simulink subsystem "GCAS"  (R2023b)
settings: Solver=VariableStepAuto  StartTime=0.0  StopTime=10.0  RelTol=1e-3
undefined symbols (not defined in the file): Altitudes, faces, Latitudes, Longitudes, spacing_in_latitude, spacing_in_longitude, vertices
libraries: simulink x3, simulink_extras x1
settings Model: Creator=cyber  LastModifiedBy=cyber

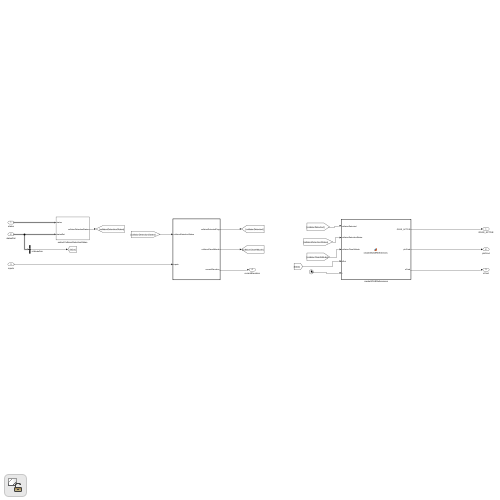
[thumbnail: Simulink's stored preview of the top-level diagram]
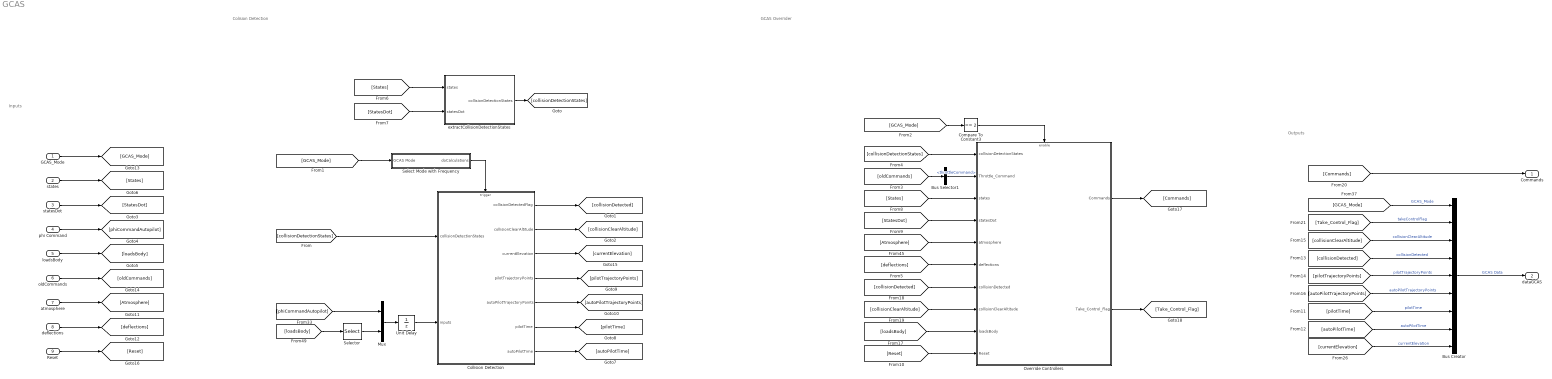
== system GCAS ==
  note: Inputs
  note: Outputs
  note: Colision Detection
  note: GCAS Overrider
  GCAS_Mode : Inport
  states : Inport  Port=2
  statesDot : Inport  Port=3
  phi Command : Inport  Port=4
  loadsBody : Inport  Port=5
  oldCommands : Inport  Port=6
  atmosphere : Inport  Port=7
  deflections : Inport  Port=8
  Reset : Inport  Port=9
  Bus Creator : BusCreator  Inputs=9
  Bus Selector1 : BusSelector  OutputSignals=throttleCommand
  Collision Detection : Subsystem  TreatAsAtomicUnit=on  SystemSampleTime=0.5
  Compare To Constant3 : simulink/Logic and Bit Operations/Compare To Constant  relop===  const=2  OutDataTypeStr=boolean
  Mux : Mux  Inputs=2
  Override Controllers : Subsystem
  Select Mode with Frequency : Subsystem
  Selector : Selector  InputPortWidth=3  IndexOptions=Index vector (dialog)  Indices=[3]  OutputSizes=1
  Unit Delay : UnitDelay  InitialCondition=[0,1]  SampleTime=-1  HasFrameUpgradeWarning=on
  extractCollisionDetectionStates : Subsystem
  Commands : Outport
  dataGCAS : Outport  Port=2
  wires:
  extractCollisionDetectionStates/1(collisionDetectionStates) -> [collisionDetectionStates]
  [collisionDetectionStates] -> Collision Detection/1(collisionDetectionStates)
  Collision Detection/1(collisionDetectedFlag) -> [collisionDetected]
  Collision Detection/2(collisionClearAltitude) -> [collisionClearAltitude]
  Collision Detection/3(currentElevation) -> [currentElevation]
  Collision Detection/4(pilotTrajectoryPoints) -> [pilotTrajectoryPoints]
  Collision Detection/5(autoPilotTrajectoryPoints) -> [autoPilotTrajectoryPoints]
  Collision Detection/7(autoPilotTime) -> [autoPilotTime]
  Collision Detection/6(pilotTime) -> [pilotTime]
  Unit Delay/1 -> Collision Detection/2(inputs)
  Mux/1 -> Unit Delay/1
  [phiCommandAutopilot] -> Mux/1
  [loadsBody] -> Selector/1
  Selector/1 -> Mux/2
  phi Command/1 -> [phiCommandAutopilot]
  loadsBody/1 -> [loadsBody]
  GCAS_Mode/1 -> [GCAS_Mode]
  oldCommands/1 -> [oldCommands]
  Override Controllers/1(Commands) -> [Commands]
  [GCAS_Mode] -> Compare To Constant3/1
  Compare To Constant3/1 -> Override Controllers/Enable
  [oldCommands] -> Bus Selector1/1
  Bus Selector1/1 -> Override Controllers/2(Throttle_Command)  "<throttleCommand>"
  [collisionDetectionStates] -> Override Controllers/1(collisionDetectionStates)
  states/1 -> [States]
  statesDot/1 -> [StatesDot]
  [States] -> extractCollisionDetectionStates/1(states)
  [StatesDot] -> extractCollisionDetectionStates/2(statesDot)
  [States] -> Override Controllers/3(states)
  [StatesDot] -> Override Controllers/4(statesDot)
  atmosphere/1 -> [Atmosphere]
  [Atmosphere] -> Override Controllers/5(atmosphere)
  Reset/1 -> [Reset]
  deflections/1 -> [deflections]
  [Reset] -> Override Controllers/10(Reset)
  [deflections] -> Override Controllers/6(deflections)
  [pilotTrajectoryPoints] -> Bus Creator/5  "pilotTrajectoryPoints"
  [Take_Control_Flag] -> Bus Creator/2  "takeControlFlag"
  [autoPilotTrajectoryPoints] -> Bus Creator/6  "autoPilotTrajectoryPoints"
  [collisionClearAltitude] -> Bus Creator/3  "collisionClearAltitude"
  [pilotTime] -> Bus Creator/7  "pilotTime"
  [currentElevation] -> Bus Creator/9  "currentElevation"
  [autoPilotTime] -> Bus Creator/8  "autoPilotTime"
  [collisionDetected] -> Bus Creator/4  "collisionDetected"
  Bus Creator/1 -> dataGCAS/1  "GCAS Data"
  [GCAS_Mode] -> Bus Creator/1  "GCAS_Mode"
  [collisionDetected] -> Override Controllers/7(collisionDetected)
  [collisionClearAltitude] -> Override Controllers/8(collisionClearAltitude)
  [Commands] -> Commands/1
  Override Controllers/2(Take_Control_Flag) -> [Take_Control_Flag]
  [loadsBody] -> Override Controllers/9(loadsBody)
  [GCAS_Mode] -> Select Mode with Frequency/1(GCAS Mode)
  Select Mode with Frequency/1(doCalculations) -> Collision Detection/Trigger

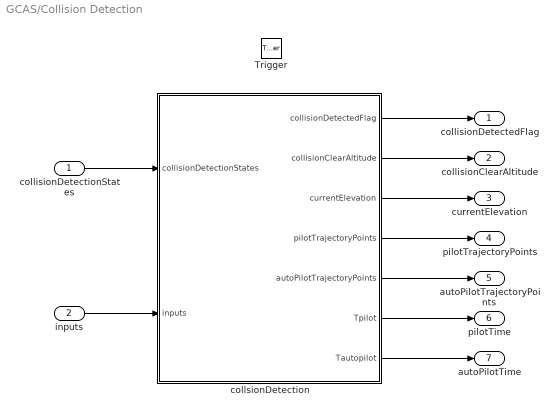
== system GCAS/Collision Detection ==
  collisionDetectionStates : Inport
  inputs : Inport  Port=2
  Trigger : TriggerPort  VariantControl=(inherit)  InitialTriggerSignalState=zero  PortDimensions=1
  collsionDetection : MATLAB Function  TreatAsAtomicUnit=on
  collisionDetectedFlag : Outport
  collisionClearAltitude : Outport  Port=2
  currentElevation : Outport  Port=3
  pilotTrajectoryPoints : Outport  Port=4
  autoPilotTrajectoryPoints : Outport  Port=5
  pilotTime : Outport  Port=6
  autoPilotTime : Outport  Port=7
  wires:
  collsionDetection/6(Tpilot) -> pilotTime/1
  collsionDetection/7(Tautopilot) -> autoPilotTime/1
  collsionDetection/5(autoPilotTrajectoryPoints) -> autoPilotTrajectoryPoints/1
  collsionDetection/4(pilotTrajectoryPoints) -> pilotTrajectoryPoints/1
  collsionDetection/3(currentElevation) -> currentElevation/1
  inputs/1 -> collsionDetection/2(inputs)
  collsionDetection/2(collisionClearAltitude) -> collisionClearAltitude/1
  collisionDetectionStates/1 -> collsionDetection/1(collisionDetectionStates)
  collsionDetection/1(collisionDetectedFlag) -> collisionDetectedFlag/1

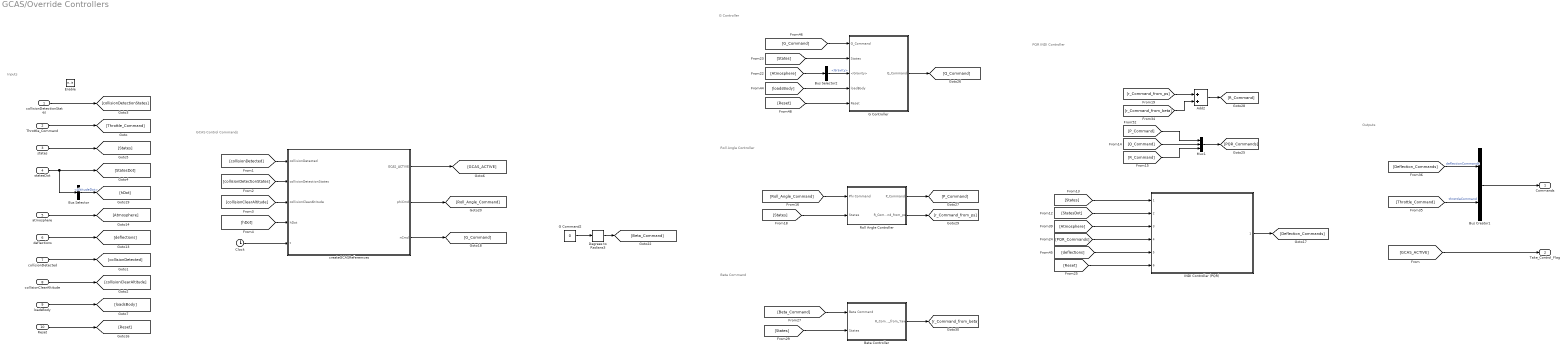
== system GCAS/Override Controllers ==
  note: Inputs
  note: Beta Command
  note: PQR INDI Controller
  note: Roll Angle Controller
  note: G Controller
  note: GCAS Control Commands
  note: Outputs
  collisionDetectionStates : Inport
  Throttle_Command : Inport  Port=2
  states : Inport  Port=3
  statesDot : Inport  Port=4
  atmosphere : Inport  Port=5
  deflections : Inport  Port=6
  collisionDetected : Inport  Port=7
  collisionClearAltitude : Inport  Port=8
  loadsBody : Inport  Port=9
  Reset : Inport  Port=10
  Enable : EnablePort
  Add2 : Sum
  Beta Controller : Subsystem  TreatAsAtomicUnit=on
  Bus Creator1 : BusCreator  Inputs=2
  Bus Selector : BusSelector  OutputSignals=AltitudeDot
  Bus Selector2 : BusSelector  OutputSignals=Gravity
  Clock : Clock
  Degrees to Radians3 : simulink_extras/Transformations/Degrees to Radians
  G Command2 : Constant  Value=0
  G Controller : Subsystem  TreatAsAtomicUnit=on
  INDI Controller (PQR) : Subsystem  ReferencedSubsystem=INDI_Controller_PQR
  Mux1 : Mux  Inputs=3
  Roll Angle Controller : Subsystem  TreatAsAtomicUnit=on
  createGCASReferemces : MATLAB Function  TreatAsAtomicUnit=on
  Commands : Outport
  Take_Control_Flag : Outport  Port=2
  wires:
  loadsBody/1 -> [loadsBody]
  [GCAS_ACTIVE] -> Take_Control_Flag/1
  collisionClearAltitude/1 -> [collisionClearAltitude]
  collisionDetected/1 -> [collisionDetected]
  Bus Selector/1 -> [hDot]  "<AltitudeDot>"
  deflections/1 -> [deflections]
  Reset/1 -> [Reset]
  atmosphere/1 -> [Atmosphere]
  states/1 -> [States]
  statesDot/1 -> Bus Selector/1, [StatesDot]
  collisionDetectionStates/1 -> [collisionDetectionStates]
  Throttle_Command/1 -> [Throttle_Command]
  createGCASReferemces/2(phiCmd) -> [Roll_Angle_Command]
  [r_Command_from_ps] -> Add2/1
  [States] -> Beta Controller/2(States)
  [Atmosphere] -> INDI Controller (PQR)/3
  Degrees to Radians3/1 -> [Beta_Command]
  G Command2/1 -> Degrees to Radians3/1
  [PQR_Commands] -> INDI Controller (PQR)/4
  [G_Command] -> G Controller/1(G_Command)
  [r_Command_from_beta] -> Add2/2
  [R_Command] -> Mux1/3
  [States] -> INDI Controller (PQR)/1
  [States] -> G Controller/2(States)
  [P_Command] -> Mux1/1
  [Beta_Command] -> Beta Controller/1(Beta Command)
  [collisionDetectionStates] -> createGCASReferemces/2(collisionDetectionStates)
  G Controller/1(Q_Command) -> [Q_Command]
  Beta Controller/1(R_Command_from_Yaw) -> [r_Command_from_beta]
  Add2/1 -> [R_Command]
  INDI Controller (PQR)/1 -> [Deflection_Commands]
  [Q_Command] -> Mux1/2
  [Atmosphere] -> Bus Selector2/1
  Roll Angle Controller/2(R_Command_from_ps) -> [r_Command_from_ps]
  Bus Selector2/1 -> G Controller/3(<Gravity>)  "<Gravity>"
  [hDot] -> createGCASReferemces/4(hDot)
  Mux1/1 -> [PQR_Commands]
  [collisionDetected] -> createGCASReferemces/1(collisionDetected)
  createGCASReferemces/1(GCAS_ACTIVE) -> [GCAS_ACTIVE]
  createGCASReferemces/3(nCmd) -> [G_Command]
  [loadsBody] -> G Controller/4(loadBody)
  [deflections] -> INDI Controller (PQR)/5
  [Deflection_Commands] -> Bus Creator1/1  "deflectionCommands"
  [Reset] -> INDI Controller (PQR)/6
  Roll Angle Controller/1(P_Command) -> [P_Command]
  [Reset] -> G Controller/5(Reset)
  [States] -> Roll Angle Controller/2(States)
  [collisionClearAltitude] -> createGCASReferemces/3(collisionClearAltitude)
  [StatesDot] -> INDI Controller (PQR)/2
  [Throttle_Command] -> Bus Creator1/2  "throttleCommand"
  Clock/1 -> createGCASReferemces/5(t)
  [Roll_Angle_Command] -> Roll Angle Controller/1(Phi Command)
  Bus Creator1/1 -> Commands/1

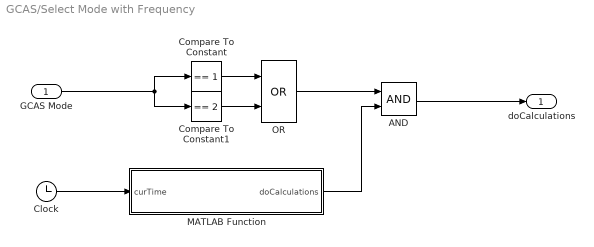
== system GCAS/Select Mode with Frequency ==
  GCAS Mode : Inport
  AND : Logic  AllPortsSameDT=off  OutDataTypeStr=boolean
  Clock : Clock
  Compare To Constant : simulink/Logic and Bit Operations/Compare To Constant  relop===  const=1  OutDataTypeStr=boolean
  Compare To Constant1 : simulink/Logic and Bit Operations/Compare To Constant  relop===  const=2  OutDataTypeStr=boolean
  MATLAB Function : MATLAB Function  TreatAsAtomicUnit=on
  OR : Logic  Operator=OR  AllPortsSameDT=off  OutDataTypeStr=boolean
  doCalculations : Outport
  wires:
  MATLAB Function/1(doCalculations) -> AND/2
  Clock/1 -> MATLAB Function/1(curTime)
  AND/1 -> doCalculations/1
  OR/1 -> AND/1
  GCAS Mode/1 -> Compare To Constant1/1, Compare To Constant/1
  Compare To Constant/1 -> OR/1
  Compare To Constant1/1 -> OR/2

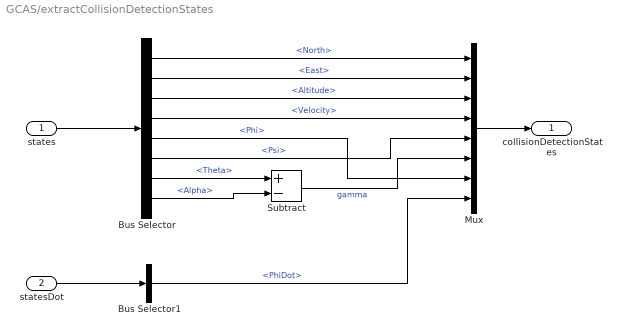
== system GCAS/extractCollisionDetectionStates ==
  states : Inport
  statesDot : Inport  Port=2
  Bus Selector : BusSelector  OutputSignals=North,East,Altitude,Velocity,Phi,Psi,Theta,Alpha
  Bus Selector1 : BusSelector  OutputSignals=PhiDot
  Mux : Mux  Inputs=8
  Subtract : Sum  Inputs=+-
  collisionDetectionStates : Outport
  wires:
  Mux/1 -> collisionDetectionStates/1
  Subtract/1 -> Mux/6  "gamma"
  Bus Selector/4 -> Mux/4  "<Velocity>"
  Bus Selector/2 -> Mux/2  "<East>"
  states/1 -> Bus Selector/1
  Bus Selector1/1 -> Mux/8  "<PhiDot>"
  Bus Selector/6 -> Mux/5  "<Psi>"
  Bus Selector/8 -> Subtract/2  "<Alpha>"
  statesDot/1 -> Bus Selector1/1
  Bus Selector/5 -> Mux/7  "<Phi>"
  Bus Selector/3 -> Mux/3  "<Altitude>"
  Bus Selector/1 -> Mux/1  "<North>"
  Bus Selector/7 -> Subtract/1  "<Theta>"

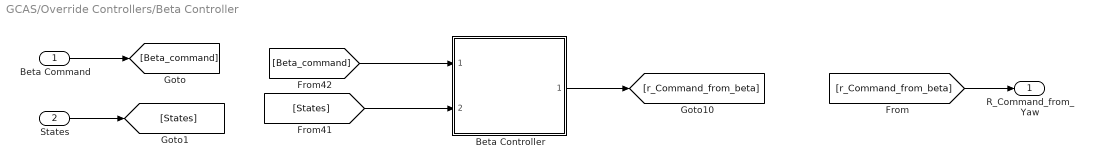
== system GCAS/Override Controllers/Beta Controller ==
  Beta Command : Inport
  States : Inport  Port=2
  Beta Controller : Subsystem  ReferencedSubsystem=Beta_Controller
  R_Command_from_Yaw : Outport
  wires:
  Beta Controller/1 -> [r_Command_from_beta]
  [States] -> Beta Controller/2
  [Beta_command] -> Beta Controller/1
  Beta Command/1 -> [Beta_command]
  [r_Command_from_beta] -> R_Command_from_Yaw/1
  States/1 -> [States]

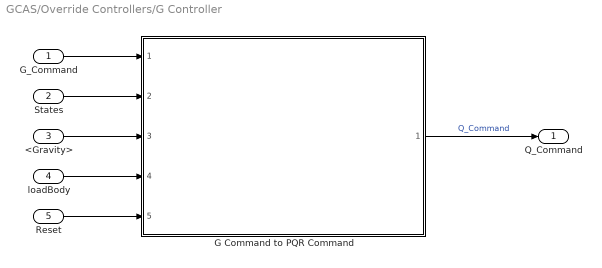
== system GCAS/Override Controllers/G Controller ==
  G_Command : Inport
  States : Inport  Port=2
  <Gravity> : Inport  Port=3
  loadBody : Inport  Port=4
  Reset : Inport  Port=5
  G Command to PQR Command : Subsystem  ReferencedSubsystem=G_Command_to_PQR_Command
  Q_Command : Outport
  wires:
  Reset/1 -> G Command to PQR Command/5
  States/1 -> G Command to PQR Command/2
  G_Command/1 -> G Command to PQR Command/1
  <Gravity>/1 -> G Command to PQR Command/3
  loadBody/1 -> G Command to PQR Command/4
  G Command to PQR Command/1 -> Q_Command/1  "Q_Command"

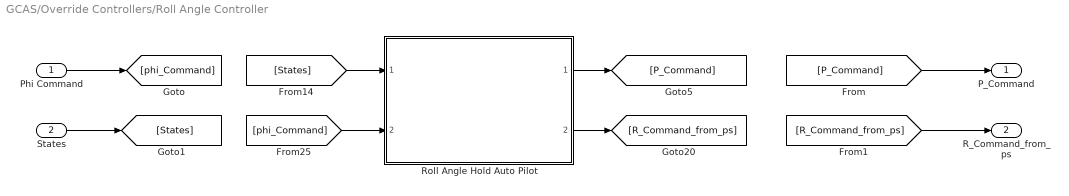
== system GCAS/Override Controllers/Roll Angle Controller ==
  Phi Command : Inport
  States : Inport  Port=2
  "Roll Angle Hold Auto Pilot " : Subsystem  ReferencedSubsystem=Roll_Angle_Hold_Auto_Pilot
  P_Command : Outport
  R_Command_from_ps : Outport  Port=2
  wires:
  States/1 -> [States]
  [R_Command_from_ps] -> R_Command_from_ps/1
  [P_Command] -> P_Command/1
  Phi Command/1 -> [phi_Command]
  [States] -> "Roll Angle Hold Auto Pilot "/1
  [phi_Command] -> "Roll Angle Hold Auto Pilot "/2
  "Roll Angle Hold Auto Pilot "/1 -> [P_Command]
  "Roll Angle Hold Auto Pilot "/2 -> [R_Command_from_ps]

== matlab function GCAS/Collision Detection/collsionDetection ==
  data: collisionDetectionStates input; collisionDetectedFlag output size=1; inputs input; Latitudes parameter; Longitudes parameter; Altitudes parameter; spacing_in_latitude parameter; spacing_in_longitude parameter; vertices parameter; faces parameter; collisionClearAltitude output; currentElevation output; pilotTrajectoryPoints output; autoPilotTrajectoryPoints output; Tpilot output; Tautopilot output
function [collisionDetectedFlag,collisionClearAltitude, currentElevation, pilotTrajectoryPoints, autoPilotTrajectoryPoints, Tpilot,Tautopilot]  = collisionDetection(collisionDetectionStates, inputs, Latitudes, Longitudes, Altitudes, spacing_in_latitude, spacing_in_longitude, vertices, faces)
    
    coder.extrinsic("visualizeTraj")
    visualize_traj = false;
    x = collisionDetectionStates(1); 
    y = collisionDetectionStates(2); 
    h = collisionDetectionStates(3);
    V = collisionDetectionStates(4);
    psi = collisionDetectionStates(5); 
    gamma = collisionDetectionStates(6); 
    phi = collisionDetectionStates(7);
    phiDot = collisionDetectionStates(8); 
    
    phiPilot = inputs(1); 
    nGPilot = inputs(2);
    Tpilot = 1;
    
    % define reference latitude longitude altitude
    lat0 = 41.10068727249253;
    lon0 = 29.024573561608477;
    h0 = 0;

    g = 9.81; % gravitational constant
    dt = 0.1; 
    T = 20;
    ts = 2.25; % Roll dynamics settling time
    OS = 1.4030 / 100; % Roll dynamics overshoot value
    zeta = - log(OS) / sqrt(pi^2+ log(OS)^2); % roll dynamics damping ratio
    wn = 4/(zeta*ts); % roll dynamics natural freq
    tsG = 2.0; % G controller settling time
    zetaG = 1; % G controller dampling ratio
    wnG = 4 / (zetaG*tsG); % G controller natural frequency

    N = floor(T/dt);
    t_array = 0:dt:T;
    states_list = zeros(N+1, 6);
    inputs_list = zeros(N+1,2);
    states_list(1,:) = [x,y,h,psi, gamma, phi];
    inputs_list(1,:) = [phiPilot, nGPilot];
    phiCmd = phiPilot;
    nGCmd = nGPilot;
    nG = nGCmd;
    nGDot = 0;
    Tautopilot = T - Tpilot;
    pilotN = floor(Tpilot/dt)-1;
    pilotTrajectoryPoints = zeros(pilotN,3);
    autoPilotN = N - pilotN;
    autoPilotTrajectoryPoints = zeros(autoPilotN,3);
    pilotNCount = 0;
    autoPilotNCount = 0;
    for i=1:N
        t = t_array(i+1);
        wingsLevelCond = abs(phi) < deg2rad(5); 
        rollRateCond = abs(phiDot) < deg2rad(5);
        if t < Tpilot
            
            % use pilots references for Tpilot period
            nGCmd = nGPilot;
            phiCmd = phiPilot;

            pilotNCount = pilotNCount + 1;
            pilotTrajectoryPoints(pilotNCount,:) = [x,y,-h];
        else
            phiCmd = 0;
            if (wingsLevelCond && rollRateCond)
                nGCmd = 5;
            else
                nG = 1 / cos(phi);
            end
            autoPilotNCount = autoPilotNCount + 1;
            autoPilotTrajectoryPoints(autoPilotNCount ,:) = [x,y,-h];
        end
        
        % add controlled roll angle dynamics
        phiDot = phiDot + dt * (phiCmd - 2*zeta*wn*phiDot - wn^2 * phi);
        phi = phi + dt * phiDot;
        nGDot = nGDot + dt * (nGCmd - 2*zetaG*wnG*nGDot - wnG^2*nG);
        nG = nG + dt*nGDot;
        % integrate equations with euler integration
        x = x + dt * V * cos(psi) * cos(gamma); % x position
        y = y + dt * V * sin(psi) * cos(gamma); % y position
        h = h + dt * V * sin(gamma); % altitude
        psi = psi + dt * g * nG /V * sin(phi) / cos(gamma); % Yaw angle
        gamma = gamma + dt * g / V *(nG *cos(phi) - cos(gamma)); % flight path angle
        states_list(i+1,:) = [x,y,h,psi, gamma, phi];
        inputs_list(i+1, :) = [phiCmd, nG];
    end
    
    x_array = states_list(:,1);
    y_array = states_list(:,2);
    h_array = states_list(:,3);
    ellipsoid = wgs84Ellipsoid(); % define Earth ellipsoid for coordinate transformation
    [pLats, pLons, pAlts] = ned2geodetic(x_array, y_array, -h_array, lat0, lon0, h0,  ellipsoid); % convert cartesian coordinates to LLA

    
    % slice states for faster interpolation
    iLat = floor((pLats(1) - Latitudes(1))/spacing_in_latitude);
    iLon = floor((pLons(1) - Longitudes(1))/spacing_in_longitude);
    idxRange = 100;
    slicedLat = Latitudes((iLat-idxRange):(iLat+idxRange));
    slicedLon = Longitudes((iLon-idxRange):(iLon+idxRange));
    slicedAlt = Altitudes((iLon-idxRange):(iLon+idxRange), (iLat-idxRange):(iLat+idxRange));
    
    
    terrain_elevations = interp2(slicedLat, slicedLon, slicedAlt, pLats,pLons); % interpolate altitude data
    
    currentElevation = h_array(1) - terrain_elevations(1);
    if visualize_traj
        visualizeTraj(states_list, slicedLat, slicedLon, slicedAlt', lat0, lon0, 0, vertices, faces)
    end

    collisionCond = double(sum((pAlts<terrain_elevations))>0); % check any of the trajectory altitudes less than terrain elevation
    collisionClearAltitude = max(max(slicedAlt)) + 200;

   
    collisionDetectedFlag = collisionCond ;

== matlab function GCAS/Override Controllers/createGCASReferemces ==
  settings: updateMethod=DISCRETE
  data: GCAS_ACTIVE output; collisionDetected input; phiCmd output; collisionDetectionStates input; nCmd output; collisionClearAltitude input; hDot input; t input
function [GCAS_ACTIVE, phiCmd, nCmd]= createGCASReferences(collisionDetected, collisionDetectionStates, collisionClearAltitude, hDot, t)
    persistent tCollisionDetected; % last time when collision is detected
    if isempty(tCollisionDetected)
        tCollisionDetected = -inf;
    end

    x = collisionDetectionStates(1);
    y = collisionDetectionStates(2);
    h = collisionDetectionStates(3);
    phi = collisionDetectionStates(7);
    phi_dot = collisionDetectionStates(8);
    
    holdAlt = 0;
    if collisionDetected
        tCollisionDetected = t;
        GCAS_ACTIVE = 1;
    elseif (not(collisionDetected) && (t - tCollisionDetected  < inf)) 
        GCAS_ACTIVE = 1;
        if (t-tCollisionDetected>5) && h > collisionClearAltitude 
            % if 5 seconds passed and altitude above collision clear
            % altitude hold altitude
            holdAlt = 1;
        end
            
    else
        GCAS_ACTIVE = 0;
        tCollisionDetected = -inf;
    end

    wingsLevelCond = abs(phi) < deg2rad(5);
    rollRateCond = abs(phi_dot) < deg2rad(5);
    if GCAS_ACTIVE ==1
        if (wingsLevelCond && rollRateCond) 
            % if wings are level and roll rate close to zero start pull-up
            phiCmd = 0;
            if holdAlt
                % run PD controller for altitude hold
                nCmd = max(min(0.01*(1000 - h) + 0.05*(-hDot) +1,5),-3);
            else
                nCmd = 5;
            end
        else
            % set wings level
            phiCmd = 0;
            nCmd = 1/cos(phi);
        end
    else
        phiCmd = 0;
        nCmd = 1;
    end

== matlab function GCAS/Select Mode with Frequency/MATLAB Function ==
  data: curTime input; doCalculations output
function doCalculations = PseudoSampleTimeChange(curTime)
% persistent oldTime
% if isempty(oldTime)
%     oldTime = -inf;
% end
sampleTime = 1;
% dt = curTime - oldTime;

if (rem(curTime,sampleTime)==0)
    % oldTime = curTime;
    doCalculations = true;
else
    doCalculations = false;
end
